simulink model "MathematicalModel"  (R2024b)
settings: Solver=VariableStepAuto  StartTime=0.0  StopTime=15  RelTol=1e-3  EnableMultiTasking=on
undefined symbols (not defined in the file or in its folder): A, Cd, g, m, rho, tau, V
libraries: fl_lib x9, nesl_utility x5, simulink_extras x2, slpidlib x1, Batteriestest7_lib x1
settings Model: PacingRate=2  ExtModeTrigDuration=2  Creator=Ali  LastModifiedBy=mygoo
settings SolverCC: AutoInsertRateTranBlk=on
settings OptimizationCC: EnhancedBackFolding=on  PassReuseOutputArgsThreshold=0  MaxStackSize=64  OptimizeBlockOrder=speed  DifferentSizesBufferReuse=on
settings DebuggingCC: ParameterTunabilityLossMsg=error
settings HardwareCC: ProdBitPerPointer=32  ProdBitPerSizeT=32  ProdBitPerPtrDiffT=32  ProdLargestAtomicInteger=Long  ProdLargestAtomicFloat=Double  ProdWordSize=32  ProdHWDeviceType=ARM Compatible->ARM Cortex  UseEmbeddedCoderFeatures=off  UseSimulinkCoderFeatures=off
settings SFSimCC: MATLABDynamicMemAlloc=off
settings RTWCC: Description=Embedded Coder  SystemTargetFile=ert.tlc  HardwareBoard=Arduino Uno R4 WiFi  TemplateMakefile=ert_default_tmf  Toolchain=Arduino ARM M4  BuildConfiguration=Faster Runs  GPUComputeCapability=3.5
settings CodeAppCC: ForceParamTrailComments=on  OperatorAnnotations=on
settings ERTTargetCC: ERTCustomFileBanners=off  SupportContinuousTime=on  SupportNonInlinedSFcns=on  RemoveResetFunc=off  SupportVariableSizeSignals=on  ModelStepFunctionPrototypeControlCompliant=off  ExtModeTransport=3  ExtModeStaticAlloc=on  ExtModeAutomaticAllocSize=off  ExtModeStaticAllocSize=8192  ExtModeMexFile=ext_xcp  ExtModeIntrfLevel=Level2 - Open  InlinedParameterPlacement=Hierarchical  DynamicArrayContainerType=coder::array

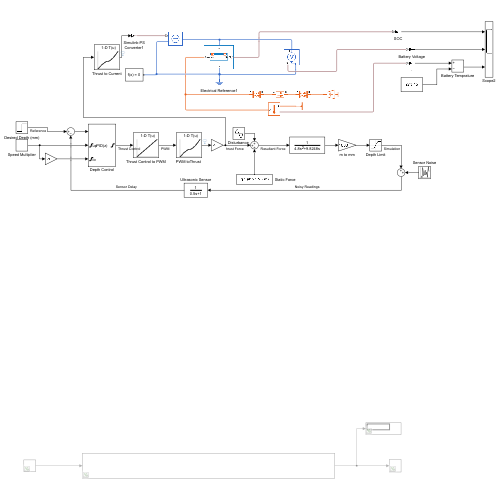
[thumbnail: Simulink's stored preview of the top-level diagram]
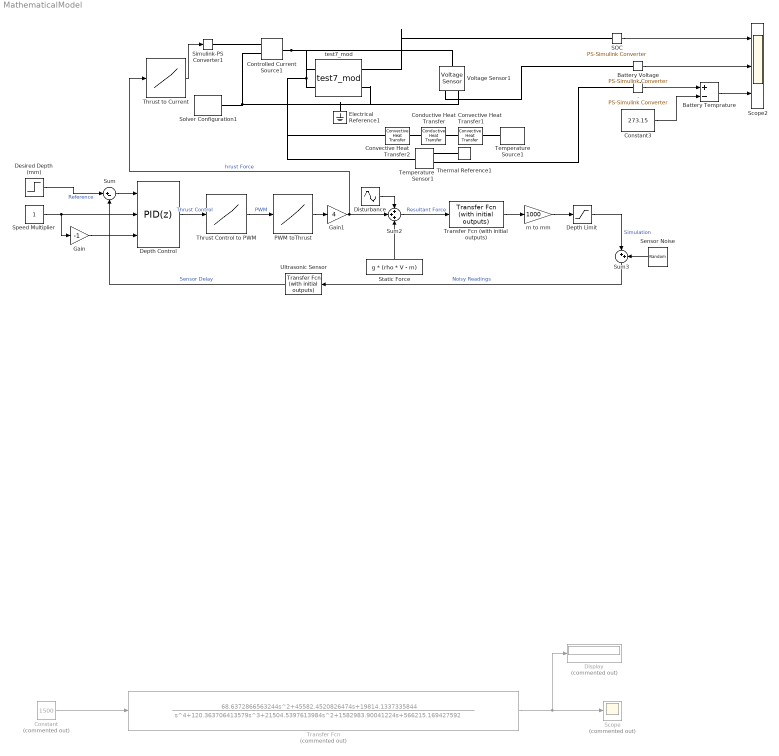
== system MathematicalModel ==
  . : nesl_utility/PS-Simulink Converter  PhysicalDomain=network_engine_domain  SubClassName=ps_output  LeftPortType=input  RightPortType=output  PseudoPeriodic=off  Frequencies=[]  VectorFormat=inherit  Unit=inherit  AffineConversion=off
  Battery Temprature : Sum  Inputs=+-
  Battery Voltage : nesl_utility/PS-Simulink Converter  PhysicalDomain=network_engine_domain  SubClassName=ps_output  LeftPortType=input  RightPortType=output  PseudoPeriodic=off  Frequencies=[]  VectorFormat=inherit  Unit=inherit  AffineConversion=off
  Conductive Heat Transfer : fl_lib/Thermal/Thermal Elements/Conductive Heat Transfer  thermal_type=foundation.enum.ConstantVariableTabulated.Constant  wall_geometry=foundation.enum.ConductionWallGeometry.Cylindrical  area=9 m^2  thickness=0.0127 m  d_in=.1016 m  d_out=.1143 m  L=0.4 m  th_cond_min=10 W/(K*m)  th_cond=0.187 W/(K*m)  th_cond_TLU=[413, 401, 392, 383, 371, 357, 342] W/(K*m)  temp_TLU=[200, 273, 400, 600, 800, 1000, 1200] K  T_specify=off  T_priority=None  T=0 K  T_nominal_specify=off  T_nominal_value=1  T_nominal_unit=K  Q_specify=off  Q_priority=None  Q=0 W  Q_nominal_specify=off  Q_nominal_value=1  Q_nominal_unit=W
  Constant : Constant  Commented=on  Value=1500
  Constant3 : Constant  Value=273.15
  Controlled Current Source1 : fl_lib/Electrical/Electrical Sources/Controlled Current Source
  Convective Heat Transfer1 : fl_lib/Thermal/Thermal Elements/Convective Heat Transfer  thermal_type=foundation.enum.constant_variable.constant  area=107160.02681 mm^2  heat_tr_coeff=50 W/(K*m^2)  min_heat_tr_coeff=1e-3 W/(K*m^2)  T_specify=off  T_priority=None  T=0 K  T_nominal_specify=off  T_nominal_value=1  T_nominal_unit=K  Q_specify=off  Q_priority=None  Q=0 W  Q_nominal_specify=off  Q_nominal_value=1  Q_nominal_unit=W
  Convective Heat Transfer2 : fl_lib/Thermal/Thermal Elements/Convective Heat Transfer  thermal_type=foundation.enum.constant_variable.constant  area=0.080246526 m^2  heat_tr_coeff=5 W/(K*m^2)  min_heat_tr_coeff=1e-3 W/(K*m^2)  T_specify=off  T_priority=None  T=0 K  T_nominal_specify=off  T_nominal_value=1  T_nominal_unit=K  Q_specify=off  Q_priority=None  Q=0 W  Q_nominal_specify=off  Q_nominal_value=1  Q_nominal_unit=W
  Depth Control : slpidlib/PID Controller  Controller=PID  Form=Parallel  TimeDomain=Discrete-time  UseExternalTs=off  SampleTime=0.0002  IntegratorMethod=Forward Euler  FilterMethod=Forward Euler  ControllerParametersSource=internal  P=33.434711290669 / 30000  I=0.0005  UseKiTs=off  D=0.0005  UseExternalDerivativeSource=off  N=1919.75319798544  UseFilter=on  TunerSelectOption=Transfer Function Based (PID Tuner App)  InitialConditionSource=internal  InitialConditionForIntegrator=0  InitialConditionForFilter=0  DifferentiatorICPrevScaledInput=0  ExternalReset=none  TrackingMode=off  Kt=1  LimitOutput=on  SatLimitsSource=external  UpperSaturationLimit=.1  LowerSaturationLimit=-.1  LinearizeAsGain=on  AntiWindupMode=none  Kb=1  LimitIntegrator=off  UpperIntegratorSaturationLimit=inf  LowerIntegratorSaturationLimit=-inf  POutMin=[]  POutMax=[]  IOutMin=[]  IOutMax=[]  DOutMin=[]  DOutMax=[]  NOutMin=[]  NOutMax=[]  SumOutMin=[]  SumOutMax=[]  SaturationOutMin=[]  SaturationOutMax=[]  PParamMin=[]  PParamMax=[]  IParamMin=[]  IParamMax=[]  DParamMin=[]  DParamMax=[]  NParamMin=[]  NParamMax=[]  KbParamMin=[]  KbParamMax=[]  KtParamMin=[]  KtParamMax=[]  KbOutMin=[]  KbOutMax=[]  KtOutMin=[]  KtOutMax=[]  IntegratorOutMin=[]  IntegratorOutMax=[]  FilterOutMin=[]  FilterOutMax=[]  SumI1OutMin=[]  SumI1OutMax=[]  SumI2OutMin=[]  SumI2OutMax=[]  SumI3OutMin=[]  SumI3OutMax=[]  SumI4OutMin=[]  SumI4OutMax=[]  SumDOutMin=[]  SumDOutMax=[]  DifferentiatorOutMin=[]  DifferentiatorOutMax=[]  FilterDiffOutCoefMin=[]  FilterDiffOutCoefMax=[]  ReciprocalOutMin=[]  ReciprocalOutMax=[]  SumDenOutMin=[]  SumDenOutMax=[]  SumNumOutMin=[]  SumNumOutMax=[]  DivideOutMin=[]  DivideOutMax=[]  UdiffTsProdOutMin=[]  UdiffTsProdOutMax=[]  NTsProdOutMin=[]  NTsProdOutMax=[]  UintegralTsProdOutMin=[]  UintegralTsProdOutMax=[]  UngainTsProdOutMin=[]  UngainTsProdOutMax=[]  ClampingZeroOutDataTypeStr=Inherit: Inherit via back propagation  ClampingZeroOutMin=[]  ClampingZeroOutMax=[]  FilterDenConstantOutDataTypeStr=Inherit: Inherit via back propagation  FilterDenConstantOutMin=[]  FilterDenConstantOutMax=[]  PCopyOutDataTypeStr=Inherit: Inherit via back propagation  PCopyOutMin=[]  PCopyOutMax=[]  NCopyOutDataTypeStr=Inherit: Inherit via back propagation  NCopyOutMin=[]  NCopyOutMax=[]  IntegratorContinuousStateAttributes=''  IntegratorStateMustResolveToSignalObject=off  IntegratorRTWStateStorageClass=Auto  FilterContinuousStateAttributes=''  FilterStateMustResolveToSignalObject=off  FilterRTWStateStorageClass=Auto  ParallelPVariant=InternalParameters  IdealPVariant=Disabled  IVariant=InternalParameters  DVariant=InternalParameters  IntegratorVariant=Discrete  SatVariant=External  AWVariant=Passthrough  PCopyVariant=Disabled  TRVariant=Disabled  FdbkBlocksVariant=Forward  IdealPFdbkVariant=Disabled  SatFdbkVariant=Disabled  DerivativeFilterVariant=ForwardEulerFilter  NVariant=InternalParameters  NCopyVariant=Disabled  FilterICVariant=InternalICsFilter  IntegratorICVariant=InternalICs  ExternalResetVariant=Disabled  TRSumVariant=Passthrough  SumFdbkVariant=Disabled  SumVariant=Sum_PID  TsampFilterVariant=InternalTs  TsampNgainVariant=Passthrough  TsampIntegralVariant=Disabled_SignalSpec  ExternalSaturationOutDataTypeStr=Inherit: Same as second input  DerivativeSourceVariant=ErrorSignal  PreIntVariant=InternalPreInt
  Depth Limit : Saturate  UpperLimit=Inf  LowerLimit=300
  Desired Depth (mm) : Step  Time=15  Before=500  After=800  SampleTime=0
  Display : Display  Commented=on
  "Disturbance " : Sin  Amplitude=.25  SampleTime=0
  Electrical Reference1 : fl_lib/Electrical/Electrical Elements/Electrical Reference
  Gain : Gain  Gain=-1
  Gain1 : Gain  Gain=4
  "PWM toThrust " : Lookup_n-D  NumberOfTableDimensions=1  BreakpointsForDimension1=[1100;1104;1108;1112;1116;1120;1124;1128;1132;1136;1140;1144;1148;1152;1156;1160;1164;1168;1172;1176;1180;1184;1188;1192;1196;1200;1204;1208;1212;1216;1220;1224;1228;1232;1236;1240;1244;1248;1252;1256;1260;1264;1268;1272;1276;1280;1284;1288;1292;1296;1300;1304;1308;1312;1316;1320;1324;1328;1332;1336;1340;1344;1348;1352;1356;1360;1364;1368;1372;1376;1380;1384;1388;1392;1396;1400;1404;1408;1412;1416;1420;1424;1428;1432;1436;1440;1444;1448;1452;1456;1460;1464;1468;1472;1476;1480;1484;1488;1492;1496;1500;1504;1508;1512;1516;1520;1524;1528;1532;1536;1540;1544;1548;1552;1556;1560;1564;1568;1572;1576;1580;1584;1588;1592;1596;1600;1604;1608;1612;1616;1620;1624;1628;1632;1636;1640;1644;1648;1652;1656;1660;1664;1668;1672;1676;1680;1684;1688;1692;1696;1700;1704;1708;1712;1716;1720;1724;1728;1732;1736;1740;1744;1748;1752;1756;1760;1764;1768;1772;1776;1780;1784;1788;1792;1796;1800;1804;1808;1812;1816;1820;1824;1828;1832;1836;1840;1844;1848;1852;1856;1860;1864;1868;1872;1876;1880;1884;1888;1892;1896;1900]  Table=[-34.500300000000003;-34.307499999999997;-34.262999999999998;-33.862499999999997;-33.372999999999998;-32.928100000000001;-32.305100000000003;-31.860099999999999;-31.281700000000001;-30.792200000000001;-30.3917;-29.991199999999999;-29.4573;-28.834299999999999;-28.3003;-27.944400000000002;-27.276900000000001;-27.0989;-26.386900000000001;-25.942;-25.452500000000001;-24.785;-24.429099999999998;-24.0731;-23.6281;-23.049600000000002;-22.9161;-22.159700000000001;-21.625699999999998;-21.358699999999999;-20.7803;-20.157299999999999;-19.8903;-19.489899999999999;-18.7334;-18.555399999999999;-17.843399999999999;-17.3095;-16.8645;-16.508500000000002;-16.019100000000002;-15.485099999999999;-15.351599999999999;-14.906599999999999;-14.5061;-14.1502;-13.749700000000001;-13.4382;-12.9932;-12.5928;-12.1478;-11.7028;-11.4358;-11.035299999999999;-10.679399999999999;-10.323399999999999;-9.9674099999999992;-9.6559299999999997;-9.3444500000000001;-8.9884699999999995;-8.67699;-8.3210099999999994;-7.9205300000000003;-7.52006;-7.2530700000000001;-6.8970900000000004;-6.6746100000000004;-6.3631200000000003;-6.0961400000000001;-5.7401600000000004;-5.3841799999999997;-5.0727000000000002;-4.80572;-4.5387300000000002;-4.1827500000000004;-3.9157700000000002;-3.6487799999999999;-3.4262999999999999;-3.1148199999999999;-2.8033299999999999;-2.5363500000000001;-2.31386;-2.0468799999999998;-1.82439;-1.6019099999999999;-1.4239200000000001;-1.20143;-0.97894000000000003;-0.80095000000000005;-0.66746000000000005;-0.44496999999999998;-0.31147999999999998;0;0;0;0;0;0;0;0;0;0;0;0;0;0;0;0;0;0.44497399999999998;0.62296300000000004;0.80095300000000003;0.97894199999999998;1.2014290000000001;1.423916;1.735398;1.9578850000000001;2.224869;2.580848;2.8478319999999999;3.203811;3.55979;3.8712719999999998;4.1827529999999999;4.5387320000000004;4.894711;5.2061929999999998;5.6511670000000001;6.0961400000000001;6.3186270000000002;6.7636010000000004;7.11958;7.5200560000000003;8.0985220000000009;8.3210090000000001;8.7214860000000005;9.0329669999999993;9.4779409999999995;9.7894229999999993;10.32339;10.72387;11.213340000000001;11.7918;12.103289999999999;12.548260000000001;12.993230000000001;13.39371;13.79419;14.328150000000001;14.817629999999999;15.2181;15.75207;16.197040000000001;16.775510000000001;17.264980000000001;17.798950000000001;18.15493;18.73339;19.26736;19.667840000000002;20.468789999999998;20.780270000000002;21.18075;22.026199999999999;22.24869;22.960650000000001;23.806100000000001;24.562550000000002;25.141020000000001;25.852969999999999;26.07546;27.054400000000001;27.276890000000002;28.25583;28.7898;29.368269999999999;29.902239999999999;30.703189999999999;31.281649999999999;31.72663;32.616579999999999;32.972560000000001;33.551020000000001;34.262979999999999;34.974939999999997;35.553400000000003;36.176369999999999;36.977319999999999;37.644779999999997;38.490229999999997;39.0687;39.513669999999998;40.314619999999998;40.759599999999999;41.338059999999999;42.228009999999998;42.984459999999999;43.38494;44.23039;44.408380000000001;44.378720000000001]  InternalRulePriority=Speed  OutDataTypeStr=double  RndMeth=Simplest
  SOC : nesl_utility/PS-Simulink Converter  PhysicalDomain=network_engine_domain  SubClassName=ps_output  LeftPortType=input  RightPortType=output  PseudoPeriodic=off  Frequencies=[]  VectorFormat=inherit  Unit=inherit  AffineConversion=off
  Scope : Scope  Commented=on
  Scope2 : Scope  NumInputPorts=3
  Sensor Noise : UniformRandomNumber  Minimum=-5  Maximum=5  SampleTime=2
  Simulink-PS Converter1 : nesl_utility/Simulink-PS Converter  PhysicalDomain=network_engine_domain  SubClassName=ps_input  LeftPortType=input  RightPortType=output  PseudoPeriodic=off  Frequencies=[]  NoiseDistribution=none  NoiseParameters=[]  Unit=1  AffineConversion=off  FilteringAndDerivatives=provide  SimscapeFilterOrder=1  InputFilterTimeConstant=0.001  UdotUserProvided=0
  Solver Configuration1 : nesl_utility/Solver Configuration  PhysicalDomain=network_engine_domain  SubClassName=solver  LeftPortType=input  RightPortType=generic  Tones=[]  Harmonics=[]  SimulateNoise=off  Profile=off  UseLocalSampling=off  EnableSwitchedLinearOptims=on  FrequencyDomain=off  UseCCode=off  RelTol=0.001  AbsTol=0.001  MinStep=1e-09  ToWorkspace=off  RevertToSquareIcSolve=off  NumHomotopyIterations=100  PhasorMode=off  PhasorModeNumHarmonics=1  ConsistencySolver=NEWTON_XTOL_AFTER_FTOL  IndexReductionMethod=DerivativeReplacement  DoDC=off  ResidualTolerance=1e-09  ConsistencyTolSource=GLOBAL  ConsistencyAbsTol=0.001  ConsistencyRelTol=0.001  ConsistencyTolFactor=0.001  UseLocalSolver=off  LocalSolverChoice=NE_BACKWARD_EULER_ADVANCER  ResolveIndetEquations=on  FunctionEvalNumThread=1  LocalSolverSampleTime=0.001  DoFixedCost=off  MaxNonlinIter=3  MaxModeIter=2  ComputeImpulses=off  ImpulseIterations=2  LinearAlgebra=auto  LinearAlgebraNumThread=0  EquationFormulation=NE_TIME_EF  DelaysMemoryBudget=1024  AutomaticFiltering=on  FilteringTimeConstant=0.001  PartitionStorageMethod=AS_NEEDED  PartitionMemoryBudget=1024  PartitionMethod=ROBUST  MultibodyUseLocalSolver=off  MultibodyLocalSolverChoice=ODE1  MultibodyLocalSolverSampleTime=0.001
  Speed Multiplier : Constant
  Static Force : Constant  Value=g * (rho * V - m)
  Sum : Sum  Inputs=|+-
  Sum2 : Sum  Inputs=+++
  Sum3 : Sum  Inputs=|++
  Temperature Sensor1 : fl_lib/Thermal/Thermal Sensors/Temperature Sensor  temperature_measure=foundation.enum.MeasurementReference.difference
  Temperature Source1 : fl_lib/Thermal/Thermal Sources/Temperature Source  temperature=25 degC
  Thermal Reference1 : fl_lib/Thermal/Thermal Elements/Thermal Reference
  Thrust Control to PWM : Lookup_n-D  NumberOfTableDimensions=1  BreakpointsForDimension1=[-1:0.01:1]  Table=1500 + 400 * ([-1:0.01:1])  InternalRulePriority=Speed  RndMeth=Simplest
  Thrust to Current : Lookup_n-D  NumberOfTableDimensions=1  BreakpointsForDimension1=[1100;1104;1108;1112;1116;1120;1124;1128;1132;1136;1140;1144;1148;1152;1156;1160;1164;1168;1172;1176;1180;1184;1188;1192;1196;1200;1204;1208;1212;1216;1220;1224;1228;1232;1236;1240;1244;1248;1252;1256;1260;1264;1268;1272;1276;1280;1284;1288;1292;1296;1300;1304;1308;1312;1316;1320;1324;1328;1332;1336;1340;1344;1348;1352;1356;1360;1364;1368;1372;1376;1380;1384;1388;1392;1396;1400;1404;1408;1412;1416;1420;1424;1428;1432;1436;1440;1444;1448;1452;1456;1460;1464;1468;1472;1476;1480;1484;1488;1492;1496;1500;1504;1508;1512;1516;1520;1524;1528;1532;1536;1540;1544;1548;1552;1556;1560;1564;1568;1572;1576;1580;1584;1588;1592;1596;1600;1604;1608;1612;1616;1620;1624;1628;1632;1636;1640;1644;1648;1652;1656;1660;1664;1668;1672;1676;1680;1684;1688;1692;1696;1700;1704;1708;1712;1716;1720;1724;1728;1732;1736;1740;1744;1748;1752;1756;1760;1764;1768;1772;1776;1780;1784;1788;1792;1796;1800;1804;1808;1812;1816;1820;1824;1828;1832;1836;1840;1844;1848;1852;1856;1860;1864;1868;1872;1876;1880;1884;1888;1892;1896;1900]  Table=[-34.500300000000003;-34.307499999999997;-34.262999999999998;-33.862499999999997;-33.372999999999998;-32.928100000000001;-32.305100000000003;-31.860099999999999;-31.281700000000001;-30.792200000000001;-30.3917;-29.991199999999999;-29.4573;-28.834299999999999;-28.3003;-27.944400000000002;-27.276900000000001;-27.0989;-26.386900000000001;-25.942;-25.452500000000001;-24.785;-24.429099999999998;-24.0731;-23.6281;-23.049600000000002;-22.9161;-22.159700000000001;-21.625699999999998;-21.358699999999999;-20.7803;-20.157299999999999;-19.8903;-19.489899999999999;-18.7334;-18.555399999999999;-17.843399999999999;-17.3095;-16.8645;-16.508500000000002;-16.019100000000002;-15.485099999999999;-15.351599999999999;-14.906599999999999;-14.5061;-14.1502;-13.749700000000001;-13.4382;-12.9932;-12.5928;-12.1478;-11.7028;-11.4358;-11.035299999999999;-10.679399999999999;-10.323399999999999;-9.9674099999999992;-9.6559299999999997;-9.3444500000000001;-8.9884699999999995;-8.67699;-8.3210099999999994;-7.9205300000000003;-7.52006;-7.2530700000000001;-6.8970900000000004;-6.6746100000000004;-6.3631200000000003;-6.0961400000000001;-5.7401600000000004;-5.3841799999999997;-5.0727000000000002;-4.80572;-4.5387300000000002;-4.1827500000000004;-3.9157700000000002;-3.6487799999999999;-3.4262999999999999;-3.1148199999999999;-2.8033299999999999;-2.5363500000000001;-2.31386;-2.0468799999999998;-1.82439;-1.6019099999999999;-1.4239200000000001;-1.20143;-0.97894000000000003;-0.80095000000000005;-0.66746000000000005;-0.44496999999999998;-0.31147999999999998;0;0;0;0;0;0;0;0;0;0;0;0;0;0;0;0;0;0.44497399999999998;0.62296300000000004;0.80095300000000003;0.97894199999999998;1.2014290000000001;1.423916;1.735398;1.9578850000000001;2.224869;2.580848;2.8478319999999999;3.203811;3.55979;3.8712719999999998;4.1827529999999999;4.5387320000000004;4.894711;5.2061929999999998;5.6511670000000001;6.0961400000000001;6.3186270000000002;6.7636010000000004;7.11958;7.5200560000000003;8.0985220000000009;8.3210090000000001;8.7214860000000005;9.0329669999999993;9.4779409999999995;9.7894229999999993;10.32339;10.72387;11.213340000000001;11.7918;12.103289999999999;12.548260000000001;12.993230000000001;13.39371;13.79419;14.328150000000001;14.817629999999999;15.2181;15.75207;16.197040000000001;16.775510000000001;17.264980000000001;17.798950000000001;18.15493;18.73339;19.26736;19.667840000000002;20.468789999999998;20.780270000000002;21.18075;22.026199999999999;22.24869;22.960650000000001;23.806100000000001;24.562550000000002;25.141020000000001;25.852969999999999;26.07546;27.054400000000001;27.276890000000002;28.25583;28.7898;29.368269999999999;29.902239999999999;30.703189999999999;31.281649999999999;31.72663;32.616579999999999;32.972560000000001;33.551020000000001;34.262979999999999;34.974939999999997;35.553400000000003;36.176369999999999;36.977319999999999;37.644779999999997;38.490229999999997;39.0687;39.513669999999998;40.314619999999998;40.759599999999999;41.338059999999999;42.228009999999998;42.984459999999999;43.38494;44.23039;44.408380000000001;44.378720000000001]  InternalRulePriority=Speed  OutDataTypeStr=double  RndMeth=Simplest
  Transfer Fcn : TransferFcn  Commented=on  Numerator=[68.6372866563244 45582.4520826474 19814.1337335844]  Denominator=[1 120.363706413579 21504.5397613984 1582983.90041224 566215.169427592]
  Transfer Fcn (with initial outputs) : simulink_extras/Additional Linear/Transfer Fcn (with initial outputs)  N=[1]  D=[m 0.5 * Cd * rho * A 0]  Y0=.5  U0=0
  Ultrasonic Sensor : simulink_extras/Additional Linear/Transfer Fcn (with initial outputs)  N=[1]  D="[tau  1]"  Y0=500  U0=500
  Voltage Sensor1 : fl_lib/Electrical/Electrical Sensors/Voltage Sensor
  m to mm : Gain  Gain=1000
  test7_mod : Batteriestest7_lib/test7_mod  SOC_vecCell=[0, .01, .02, .03, .04, .05, .06, .07, .08, .09, .1, .11, .12, .13, .14, .15, .16, .17, .18, .19, .2, .21, .22, .23, .24, .25, .26, .27, .28, .29, .3, .31, .32, .33, .34, .35, .36, .37, .38, .39, .4, .41, .42, .43, .44, .45, .46, .47, .48, .49, .5, .51, .52, .53, .54, .55, .56, .57, .58, .59, .6, .61, .62, .63, .64, .65, .66, .67, .68, .69, .7, .71, .72, .73, .74, .75, .76, .77, .78, .79, .8, .81, .82, .83, .84, .85, .86, .87, .88, .89, .9, .91, .92, .93, .94, .95, .96, .97, .98, .99, 1]  V0_vecCell=[2.90003, 2.94341, 2.98679, 3.04987, 3.09433, 3.12791, 3.16031, 3.20369, 3.23862, 3.26689, 3.29115, 3.31383, 3.33202, 3.35112, 3.36833, 3.38413, 3.39973, 3.41137, 3.42149, 3.43136, 3.44073, 3.45027, 3.46068, 3.47113, 3.47814, 3.48494, 3.49199, 3.49905, 3.50562, 3.51187, 3.51861, 3.52535, 3.53209, 3.53818, 3.54353, 3.54849, 3.55353, 3.55855, 3.56357, 3.56831, 3.57308, 3.57787, 3.58264, 3.58755, 3.5925, 3.5985, 3.60496, 3.61149, 3.61805, 3.6246, 3.63116, 3.63855, 3.64609, 3.65336, 3.66064, 3.66791, 3.67613, 3.68522, 3.69443, 3.70367, 3.713, 3.72241, 3.73154, 3.74037, 3.7492, 3.75786, 3.76617, 3.77556, 3.78485, 3.79413, 3.8034, 3.81149, 3.81977, 3.82804, 3.83631, 3.84472, 3.85317, 3.86155, 3.86993, 3.87831, 3.88686, 3.89534, 3.90461, 3.91454, 3.92565, 3.93721, 3.94924, 3.96155, 3.97383, 3.98598, 3.99856, 4.01117, 4.02361, 4.03609, 4.04694, 4.05695, 4.06641, 4.07551, 4.08514, 4.09447, 4.10453] V  V_rangeCell=[2.25, Inf] V  R0_vecCell=[.1741, .15823, .14313, .13285, .12044, .10641, .09605, .09162, .08758, .08349, .08021, .07738, .07487, .07338, .07189, .07117, .0704, .06898, .06755, .06631, .06509, .06388, .06326, .06281, .06182, .06095, .06025, .05955, .05877, .05807, .05761, .05714, .05668, .05611, .05546, .0549, .05439, .05388, .05337, .0528, .05223, .05165, .05106, .05046, .04986, .04945, .04913, .04883, .04854, .04826, .04797, .04782, .04765, .0473, .04695, .04661, .04638, .0463, .04625, .04621, .04624, .04628, .04628, .04623, .04617, .04599, .04573, .0457, .04568, .04565, .04563, .04535, .0451, .04486, .04461, .04446, .04435, .04423, .04411, .044, .04372, .04339, .04323, .0432, .04344, .04374, .0441, .04452, .04494, .0454, .04594, .0463, .04649, .04668, .04629, .04541, .04438, .04326, .04154, .03869, .03326] Ohm  AHCell=3.153 A*hr  extrapolation_optionCell=simscape.enum.extrapolation.nearest  thermal_massCell=44.55 J/K  AmbientResistance=25 K/W  InterCellThermalResistance=1 K/W  InterParallelAssemblyThermalResistance=1 K/W  P=5  S=4  NumInterCellThermalConnections=16  NumInterParallelAssemblyThermalConnections=39  InterParallelAssemblyConnectionsMapping=[1, 1, 1, 1, 1, 1, 1, 1, 1, 1, 1, 1, 1, 2, 2, 2, 2, 2, 2, 2, 2, 2, 2, 2, 2, 2, 3, 3, 3, 3, 3, 3, 3, 3, 3, 3, 3, 3, 3; 2, 2, 2, 2, 2, 2, 2, 2, 2, 2, 2, 2, 2, 3, 3, 3, 3, 3, 3, 3, 3, 3, 3, 3, 3, 3, 4, 4, 4, 4, 4, 4, 4, 4, 4, 4, 4, 4, 4]  InterParallelAssemblyCellConnectionsMapping=[1, 1, 2, 2, 2, 3, 3, 3, 4, 4, 4, 5, 5, 1, 1, 2, 2, 2, 3, 3, 3, 4, 4, 4, 5, 5, 1, 1, 2, 2, 2, 3, 3, 3, 4, 4, 4, 5, 5; 1, 2, 1, 2, 3, 2, 3, 4, 3, 4, 5, 4, 5, 1, 2, 1, 2, 3, 2, 3, 4, 3, 4, 5, 4, 5, 1, 2, 1, 2, 3, 2, 3, 4, 3, 4, 5, 4, 5]  InterCellConnectionsMapping=[1, 2, 3, 4, 1, 2, 3, 4, 1, 2, 3, 4, 1, 2, 3, 4; 2, 3, 4, 5, 2, 3, 4, 5, 2, 3, 4, 5, 2, 3, 4, 5]  iCell_specify=off  iCell_priority=None  iCell=repmat(0, 20, 1) A  iCell_nominal_specify=off  iCell_nominal_value=1  iCell_nominal_unit=A  vCell_specify=off  vCell_priority=None  vCell=repmat(0, 20, 1) V  vCell_nominal_specify=off  vCell_nominal_value=1  vCell_nominal_unit=V  socCell_specify=off  socCell_priority=High  socCell=repmat(1, 20, 1)  socCell_nominal_specify=off  socCell_nominal_value=1  socCell_nominal_unit=1  numCyclesCell_specify=off  numCyclesCell_priority=High  numCyclesCell=repmat(0, 20, 1)  numCyclesCell_nominal_specify=off  numCyclesCell_nominal_value=1  numCyclesCell_nominal_unit=1  temperatureCell_specify=off  temperatureCell_priority=High  temperatureCell=repmat(298.15, 20, 1) K  temperatureCell_nominal_specify=off  temperatureCell_nominal_value=1  temperatureCell_nominal_unit=K  vParallelAssembly_specify=off  vParallelAssembly_priority=None  vParallelAssembly=repmat(0, 4, 1) V  vParallelAssembly_nominal_specify=off  vParallelAssembly_nominal_value=1  vParallelAssembly_nominal_unit=V  socParallelAssembly_specify=off  socParallelAssembly_priority=None  socParallelAssembly=repmat(1, 4, 1)  socParallelAssembly_nominal_specify=off  socParallelAssembly_nominal_value=1  socParallelAssembly_nominal_unit=1
      settings: InternalSimscapePortConfiguration="{\"Bottom\":[{\"id\":\"n\",\"label\":\"-\",\"type\":\"foundation.electrical.electrical\"}],\"Left\":[{\"id\":\"AmbH\",\"label\":\"AmbH\",\"type\":\"foundation.thermal.thermal\"}],\"Right\":[{\"id\":\"socOutCell\",\"label\":\"SOC\",\"type\":\"output\"}],\"Top\":[{\"id\":\"p\",\"label\":\"+\",\"type\":\"foundation.electrical.electrical\"}]}"
  wires:
  Constant/1 -> Transfer Fcn/1
  Transfer Fcn/1 -> Scope/1, Display/1
  Sum/1 -> Depth Control/1
  Desired Depth (mm)/1 -> Sum/1  "Reference"
  Sum2/1 -> Transfer Fcn (with initial outputs)/1  "Resultant Force"
  Transfer Fcn (with initial outputs)/1 -> m to mm/1
  Depth Control/1 -> Thrust Control to PWM/1  "Thrust Control"
  Thrust Control to PWM/1 -> "PWM toThrust "/1  "PWM"
  "PWM toThrust "/1 -> Gain1/1
  Gain/1 -> Depth Control/3
  Speed Multiplier/1 -> Depth Control/2, Gain/1
  Gain1/1 -> Sum2/2, Thrust to Current/1  "hrust Force"
  Ultrasonic Sensor/1 -> Sum/2  "Sensor Delay"
  Static Force/1 -> Sum2/3
  Sum3/1 -> Ultrasonic Sensor/1  "Noisy Readings"
  m to mm/1 -> Depth Limit/1
  Depth Limit/1 -> Sum3/1  "Simulation"
  "Disturbance "/1 -> Sum2/1
  Sensor Noise/1 -> Sum3/2
  Battery Voltage/1 -> Scope2/2
  Battery Temprature/1 -> Scope2/3
  Constant3/1 -> Battery Temprature/2
  SOC/1 -> Scope2/1
  ./1 -> Battery Temprature/1
  Thrust to Current/1 -> Simulink-PS Converter1/1
  connections:
  Solver Configuration1/RConn1 -- Electrical Reference1/LConn1 -- Voltage Sensor1/RConn2 -- test7_mod/RConn2 -- Controlled Current Source1/RConn2
  test7_mod/LConn1 -- Temperature Sensor1/LConn1 -- Convective Heat Transfer2/LConn1
  Controlled Current Source1/LConn1 -- Voltage Sensor1/LConn1 -- test7_mod/LConn2
  Conductive Heat Transfer/RConn1 -- Convective Heat Transfer1/LConn1
  Thermal Reference1/LConn1 -- Temperature Sensor1/RConn1
  test7_mod/RConn1 -- SOC/LConn1
  Simulink-PS Converter1/RConn1 -- Controlled Current Source1/RConn1
  Temperature Source1/LConn1 -- Convective Heat Transfer1/RConn1
  Convective Heat Transfer2/RConn1 -- Conductive Heat Transfer/LConn1
  ./LConn1 -- Temperature Sensor1/RConn2
  Battery Voltage/LConn1 -- Voltage Sensor1/RConn1
